simulink model "MassaMolaLinearidade"  (Simulink 7.5)
settings: Solver=ode45  StartTime=0.0  StopTime=100  RelTol=1e-3
settings Model: Creator=Leonardo  LastModifiedBy=Leo

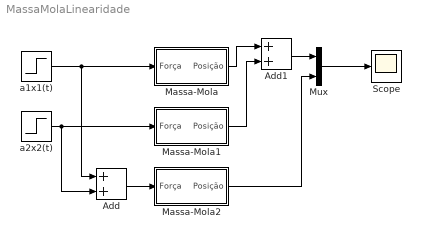
== system MassaMolaLinearidade ==
  Add : Sum  OutDataType=sfix(16)  OutScaling=2^-10
  Add1 : Sum  OutDataType=sfix(16)  OutScaling=2^-10
  Massa-Mola : Subsystem
  Massa-Mola1 : Subsystem
  Massa-Mola2 : Subsystem
  Mux : Mux  Inputs=2
  Scope : Scope
      settings: TimeRange=100  YMin=0  YMax=1
  a1x1(t) : Step  Time=0  After=20  SampleTime=0
  a2x2(t) : Step  Time=0  After=60  SampleTime=0
  wires:
  a1x1(t)/1 -> Add/1, Massa-Mola/1(Força)
  Mux/1 -> Scope/1
  a2x2(t)/1 -> Add/2, Massa-Mola1/1(Força)
  Add/1 -> Massa-Mola2/1(Força)
  Massa-Mola/1(Posição) -> Add1/1
  Massa-Mola1/1(Posição) -> Add1/2
  Add1/1 -> Mux/1
  Massa-Mola2/1(Posição) -> Mux/2

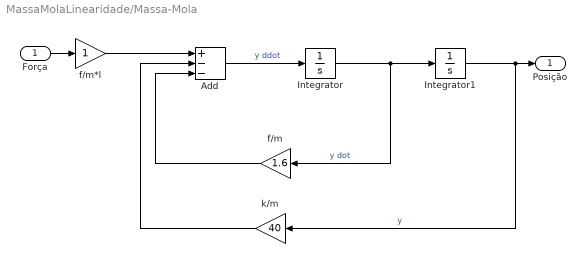
== system MassaMolaLinearidade/Massa-Mola ==
  Força : Inport
  Add : Sum  Inputs=+--
  Integrator : Integrator
  Integrator1 : Integrator
  f/m : Gain  Gain=1.6
  f/m*l : Gain
  k/m : Gain  Gain=40
  Posição : Outport
  wires:
  Integrator/1 -> Integrator1/1, f/m/1  "y dot"
  Add/1 -> Integrator/1  "y ddot"
  Integrator1/1 -> Posição/1, k/m/1  "y"
  k/m/1 -> Add/2
  f/m/1 -> Add/3
  f/m*l/1 -> Add/1
  Força/1 -> f/m*l/1

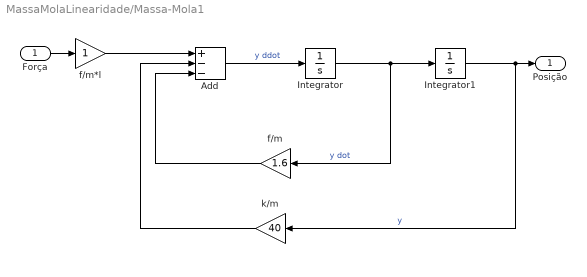
== system MassaMolaLinearidade/Massa-Mola1 ==
  Força : Inport
  Add : Sum  Inputs=+--
  Integrator : Integrator
  Integrator1 : Integrator
  f/m : Gain  Gain=1.6
  f/m*l : Gain
  k/m : Gain  Gain=40
  Posição : Outport
  wires:
  Integrator/1 -> Integrator1/1, f/m/1  "y dot"
  Add/1 -> Integrator/1  "y ddot"
  Integrator1/1 -> Posição/1, k/m/1  "y"
  k/m/1 -> Add/2
  f/m/1 -> Add/3
  f/m*l/1 -> Add/1
  Força/1 -> f/m*l/1

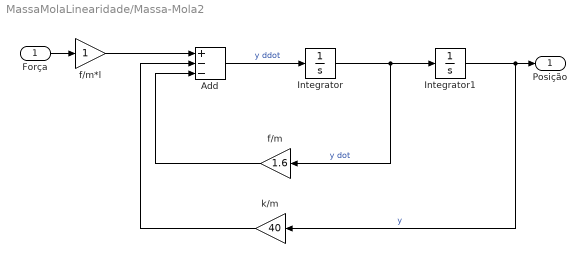
== system MassaMolaLinearidade/Massa-Mola2 ==
  Força : Inport
  Add : Sum  Inputs=+--
  Integrator : Integrator
  Integrator1 : Integrator
  f/m : Gain  Gain=1.6
  f/m*l : Gain
  k/m : Gain  Gain=40
  Posição : Outport
  wires:
  Integrator/1 -> Integrator1/1, f/m/1  "y dot"
  Add/1 -> Integrator/1  "y ddot"
  Integrator1/1 -> Posição/1, k/m/1  "y"
  k/m/1 -> Add/2
  f/m/1 -> Add/3
  f/m*l/1 -> Add/1
  Força/1 -> f/m*l/1
